simulink model "ControlR2019A"  (R2019a)
settings: Solver=FixedStepAuto  StartTime=0.0  StopTime=t_sim  FixedStep=TimeStep  RelTol=1e-3
values from neighbouring files (symbols this model uses):
  nmax = 2    [main_SCA.m]    (also in main_SCA_alt.m; main_SCA_v3.m)
  Use_IGRF = 0    [main_SCA.m]    (also in main_SCA_alt.m; main_SCA_v3.m)
undefined symbols (not defined in the file or in its folder): att, date, deg, DipoleMod, DiscIntNeverNeededParam, km, orbit, rad, s, sat
libraries: aerolibconvert2 x10, aerolibutil x10, vrlib x6, simulink x5, sharedtransform x4, dspmathops x4, sharedutil x2, dspstat3 x1, aerolibgravity2 x1, aerolibcelestial x1
(part 1 of 2)
settings Model: Creator=colpari  LastModifiedBy=colpari

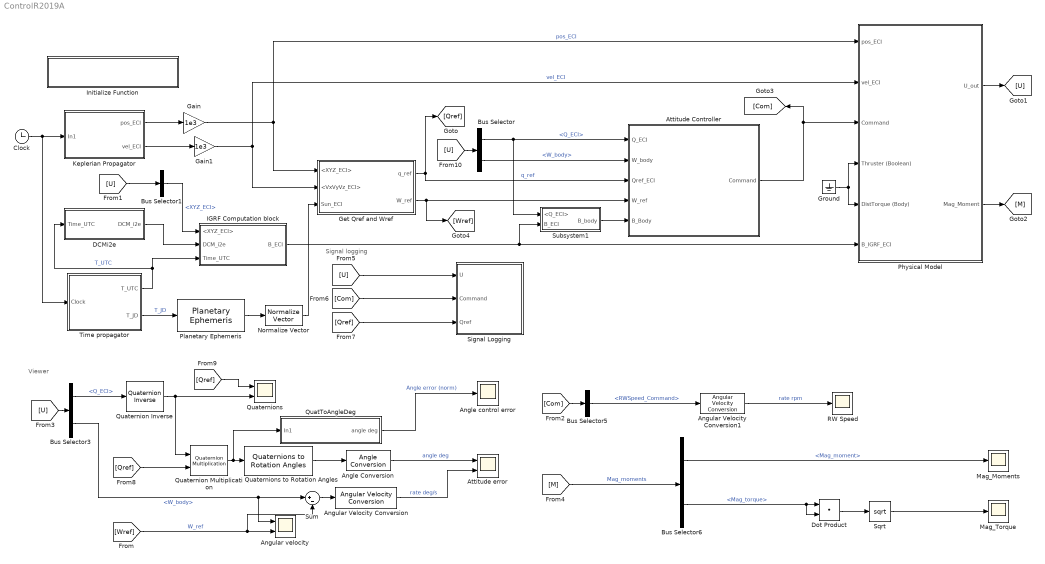
== system ControlR2019A ==
  note: Viewer
  note: Signal logging
  Angle Conversion : aerolibconvert2/Angle Conversion  IU=rad  OU=deg
  Angle control error : Scope
  Angular Velocity Conversion : aerolibconvert2/Angular Velocity Conversion  IU=rad/s  OU=deg/s
  Angular Velocity Conversion1 : aerolibconvert2/Angular Velocity Conversion  IU=rad/s  OU=rpm
  Angular velocity : Scope  NumInputPorts=2
  Attitude Controller : Subsystem  TreatAsAtomicUnit=on
  Attitude error : Scope  NumInputPorts=2
  Bus Selector : BusSelector  OutputSignals=Q_ECI,W_body
  Bus Selector1 : BusSelector  OutputSignals=XYZ_ECI
  Bus Selector3 : BusSelector  OutputSignals=Q_ECI,W_body
  Bus Selector5 : BusSelector  OutputSignals=RWSpeed_Command
  Bus Selector6 : BusSelector  OutputSignals=Mag_moment,Mag_torque
  Clock : Clock
  DCMi2e : Subsystem  TreatAsAtomicUnit=on  SystemSampleTime=1
  Dot Product : DotProduct  InputSameDT=on  OutDataTypeStr=Inherit: Inherit via internal rule
  Gain : Gain  Gain=1e3
  Gain1 : Gain  Gain=1e3
  Get Qref and Wref : Subsystem
  Ground : Ground
  IGRF Computation block : Subsystem
  Initialize Function : Subsystem  TreatAsAtomicUnit=on
  Keplerian Propagator : Subsystem
  Mag_Moments : Scope
  Mag_Torque : Scope
  Normalize Vector : vrlib/Utilities/Normalize Vector  maxzero=0
  Physical Model : Subsystem
      settings: MinAlgLoopOccurrences=on
  Planetary Ephemeris : aerolibcelestial/Planetary Ephemeris  kmflag=km,km/s  epochflag=Julian date  de=DE405  nCenter=Earth  nTarget=Sun  errorflag=Error  velflag=off
      settings: SourceProductBaseCode=AE
  QuatToAngleDeg : Subsystem
  Quaternion Inverse : aerolibutil/Quaternion Inverse
  Quaternion Multiplication : aerolibutil/Quaternion Multiplication
  Quaternions : Scope  NumInputPorts=2
  Quaternions to Rotation Angles : sharedtransform/Quaternions to Rotation Angles  rotationOrder=ZYX  aMode=aMode
      settings: SourceProductBaseCode=AE,PW,MT,UV,VE,VP
  RW Speed : Scope
  Signal Logging : Subsystem
  Sqrt : Sqrt  SaturateOnIntegerOverflow=on
  Subsystem1 : Subsystem
  Sum : Sum  Inputs=|+-
  Time propagator : Subsystem
  wires:
  Clock/1 -> Keplerian Propagator/1(In1), Time propagator/1(Clock)
  Keplerian Propagator/1(pos_ECI) -> Gain/1
  Keplerian Propagator/2(vel_ECI) -> Gain1/1
  Planetary Ephemeris/1 -> Normalize Vector/1
  Normalize Vector/1 -> Get Qref and Wref/3(Sun_ECI)
  Time propagator/2(T_JD) -> Planetary Ephemeris/1  "T_JD"
  Get Qref and Wref/1(q_ref) -> Attitude Controller/3(Qref_ECI), [Qref]  "q_ref"
  Physical Model/1(U_out) -> [U]
  Time propagator/1(T_UTC) -> DCMi2e/1(Time_UTC), IGRF Computation block/3("Time_UTC ")  "T_UTC"
  Gain/1 -> Physical Model/1(pos_ECI), Get Qref and Wref/1(<XYZ_ECI>)  "pos_ECI"
  Gain1/1 -> Physical Model/2(vel_ECI), Get Qref and Wref/2(<VxVyVz_ECI>)  "vel_ECI"
  DCMi2e/1(DCM_i2e) -> IGRF Computation block/2("DCM_i2e ")
  Attitude Controller/1(Command) -> [Com], Physical Model/3(Command)
  IGRF Computation block/1(B_ECI) -> Subsystem1/2(B_ECI), Physical Model/6(B_IGRF_ECI)
  [U] -> Bus Selector/1
  Bus Selector/1 -> Subsystem1/1(<Q_ECI>), Attitude Controller/1(Q_ECI)  "<Q_ECI>"
  Bus Selector/2 -> Attitude Controller/2(W_body)  "<W_body>"
  [U] -> Bus Selector1/1
  Bus Selector1/1 -> IGRF Computation block/1(<XYZ_ECI>)  "<XYZ_ECI>"
  [Qref] -> Signal Logging/3(Qref)
  Quaternions to Rotation Angles/1 -> Angle Conversion/1
  Bus Selector6/2 -> Dot Product/2, Dot Product/1  "<Mag_torque>"
  Bus Selector6/1 -> Mag_Moments/1  "<Mag_moment>"
  Dot Product/1 -> Sqrt/1
  Bus Selector3/1 -> Quaternion Inverse/1  "<Q_ECI>"
  Sqrt/1 -> Mag_Torque/1
  Bus Selector5/1 -> Angular Velocity Conversion1/1  "<RWSpeed_Command>"
  [Com] -> Signal Logging/2(Command)
  [Com] -> Bus Selector5/1
  Bus Selector3/2 -> Sum/1, Angular velocity/1  "<W_body>"
  [Qref] -> Quaternion Multiplication/2
  [U] -> Bus Selector3/1
  Quaternion Inverse/1 -> Quaternion Multiplication/1, Quaternions/2
  [M] -> Bus Selector6/1  "Mag_moments"
  Angular Velocity Conversion/1 -> Attitude error/2  "rate deg/s"
  Quaternion Multiplication/1 -> QuatToAngleDeg/1(In1), Quaternions to Rotation Angles/1
  [U] -> Signal Logging/1(U)
  Angle Conversion/1 -> Attitude error/1  "angle deg"
  Angular Velocity Conversion1/1 -> RW Speed/1  "rate rpm"
  Physical Model/2(Mag_Moment) -> [M]
  Subsystem1/1(B_body) -> Attitude Controller/5(B_Body)
  Ground/1 -> Physical Model/5(DistTorque (Body)), Physical Model/4(Thruster (Boolean))
  QuatToAngleDeg/1(angle deg) -> Angle control error/1  "Angle error (norm)"
  [Qref] -> Quaternions/1
  Get Qref and Wref/2(W_ref) -> [Wref], Attitude Controller/4(W_ref)
  [Wref] -> Sum/2, Angular velocity/2  "W_ref"
  Sum/1 -> Angular Velocity Conversion/1

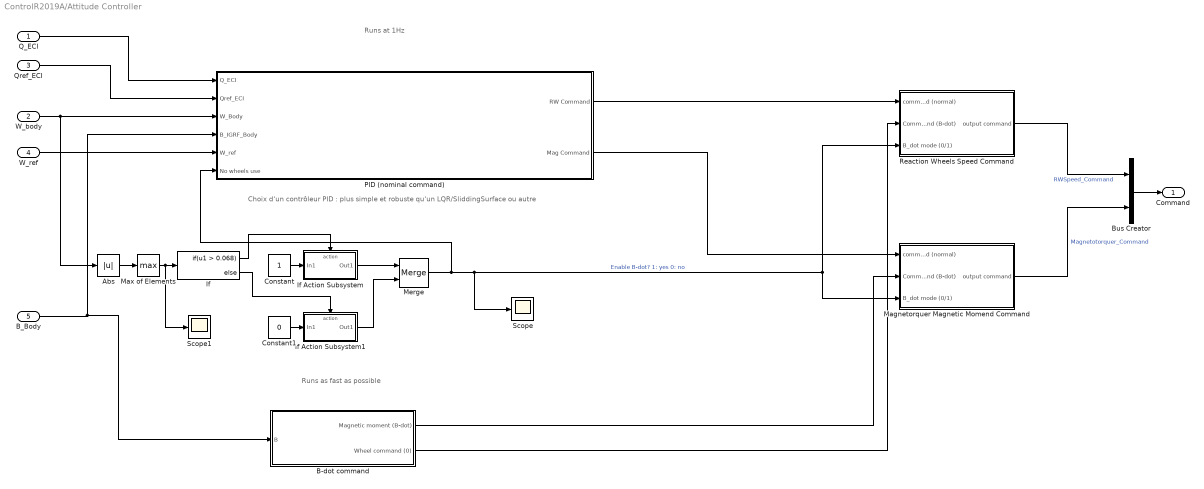
== system ControlR2019A/Attitude Controller ==
  note: Choix d'un contrôleur PID : plus simple et robuste qu'un LQR/SliddingSurface ou autre
  note: Runs as fast as possible
  note: Runs at 1Hz
  Q_ECI : Inport
  W_body : Inport  Port=2
  Qref_ECI : Inport  Port=3
  W_ref : Inport  Port=4
  B_Body : Inport  Port=5
  Abs : Abs
  B-dot command : Subsystem  TreatAsAtomicUnit=on
  Bus Creator : BusCreator  Inputs=2
  Constant : Constant
  Constant1 : Constant  Value=0
  If : If  IfExpression=u1 > 0.068
  If Action Subsystem : Subsystem  TreatAsAtomicUnit=on
  If Action Subsystem1 : Subsystem  TreatAsAtomicUnit=on
  Magnetorquer Magnetic Momend Command : Subsystem
  Max of Elements : MinMax  Function=max
  Merge : Merge
  PID (nominal command) : Subsystem  TreatAsAtomicUnit=on  SystemSampleTime=1
  Reaction Wheels Speed Command : Subsystem
  Scope : Scope
  Scope1 : Scope
  Command : Outport  VectorParamsAs1DForOutWhenUnconnected=off
  wires:
  B_Body/1 -> B-dot command/1(B), PID (nominal command)/4(B_IGRF_Body)
  Magnetorquer Magnetic Momend Command/1(output command) -> Bus Creator/2  "Magnetotorquer_Command"
  Reaction Wheels Speed Command/1(output command) -> Bus Creator/1  "RWSpeed_Command"
  B-dot command/2(Wheel command (0)) -> Reaction Wheels Speed Command/2(Command (B-dot))
  B-dot command/1(Magnetic moment (B-dot)) -> Magnetorquer Magnetic Momend Command/2(Command (B-dot))
  Q_ECI/1 -> PID (nominal command)/1(Q_ECI)
  Qref_ECI/1 -> PID (nominal command)/2(Qref_ECI)
  PID (nominal command)/1(RW Command) -> Reaction Wheels Speed Command/1(" command (normal)")
  PID (nominal command)/2(Mag Command) -> Magnetorquer Magnetic Momend Command/1(" command (normal)")
  Bus Creator/1 -> Command/1
  Abs/1 -> Max of Elements/1
  If/1 -> If Action Subsystem/Action
  If Action Subsystem1/1(Out1) -> Merge/2
  Max of Elements/1 -> Scope1/1, If/1
  If/2 -> If Action Subsystem1/Action
  If Action Subsystem/1(Out1) -> Merge/1
  Constant/1 -> If Action Subsystem/1(In1)
  Merge/1 -> Scope/1, Magnetorquer Magnetic Momend Command/3(B_dot mode (0/1)), Reaction Wheels Speed Command/3(B_dot mode (0/1)), PID (nominal command)/6(No wheels use)  "Enable B-dot? 1: yes 0: no"
  Constant1/1 -> If Action Subsystem1/1(In1)
  W_body/1 -> Abs/1, PID (nominal command)/3(W_Body)
  W_ref/1 -> PID (nominal command)/5(W_ref)

== system ControlR2019A/DCMi2e ==
  note: Slower subsytem because it's too slow
  Time_UTC : Inport
  ECI to ECEF : MATLABFcn  MATLABFcn=eci2ecef  OutputDimensions=[3;3]  Output1D=off
  DCM_i2e : Outport
  wires:
  ECI to ECEF/1 -> DCM_i2e/1
  Time_UTC/1 -> ECI to ECEF/1

== system ControlR2019A/Get Qref and Wref ==
  <XYZ_ECI> : Inport
  <VxVyVz_ECI> : Inport  Port=2
  Sun_ECI : Inport  Port=3
  Manual Switch : ManualSwitch  CurrentSetting=0
  Manual Switch1 : ManualSwitch  CurrentSetting=0
  Scope : Scope  NumInputPorts=2
  q_orbital : Subsystem
  q_sun_aero : Subsystem
  q_ref : Outport
  W_ref : Outport  Port=2
  wires:
  q_sun_aero/1(Q_sun_aero) -> Manual Switch/2
  <VxVyVz_ECI>/1 -> q_sun_aero/2(<VxVyVz_ECI>), q_orbital/2(<VxVyVz_ECI>)
  q_orbital/1(Q_orbit) -> Manual Switch/1
  Sun_ECI/1 -> q_sun_aero/1(Sun_ECI)
  <XYZ_ECI>/1 -> q_orbital/1(<XYZ_ECI>)
  Manual Switch/1 -> q_ref/1, Scope/1
  Manual Switch1/1 -> Scope/2, W_ref/1
  q_sun_aero/2(W_sun_aero) -> Manual Switch1/2
  q_orbital/2(W_orbit) -> Manual Switch1/1

== system ControlR2019A/IGRF Computation block ==
  <XYZ_ECI> : Inport
  "DCM_i2e " : Inport  Port=2
  "Time_UTC " : Inport  Port=3
  Bus Creator : BusCreator  Inputs=5
  Bus Selector4 : BusSelector  OutputSignals=XYZ_ECI
  Demux : Demux  Outputs=2
  ECI To LLA : MATLAB Function  TreatAsAtomicUnit=on
  Obtain B_ECI : Subsystem
  Product : Product  Multiplication=Matrix(*)
  Reshape : Reshape  OutputDimensionality=Row vector (2-D)
  Terminator : Terminator
  B_ECI : Outport  VectorParamsAs1DForOutWhenUnconnected=off
  wires:
  ECI To LLA/3(long) -> Bus Creator/3
  ECI To LLA/2(lat) -> Bus Creator/2
  ECI To LLA/1(h) -> Bus Creator/1
  Demux/1 -> Bus Creator/4
  Demux/2 -> Terminator/1
  "DCM_i2e "/1 -> Product/2, Bus Creator/5  "DCM_i2e"
  <XYZ_ECI>/1 -> Bus Selector4/1
  Reshape/1 -> Product/1
  Product/1 -> ECI To LLA/1(X_ECEF)
  Bus Selector4/1 -> Reshape/1  "<XYZ_ECI>"
  Bus Creator/1 -> Obtain B_ECI/1(In1)
  Obtain B_ECI/1(Out1) -> B_ECI/1
  "Time_UTC "/1 -> Demux/1

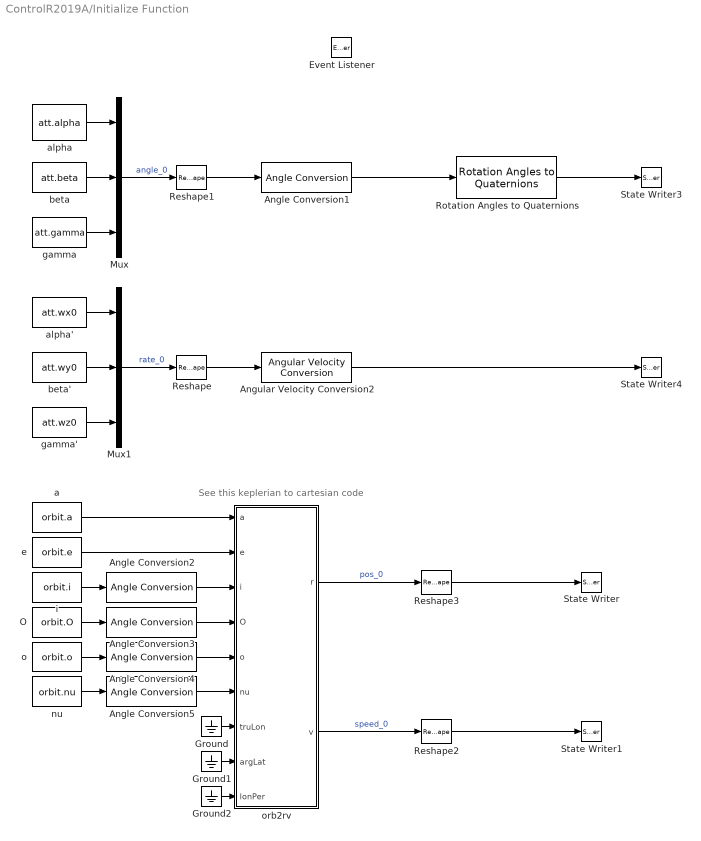
== system ControlR2019A/Initialize Function ==
  note: See this keplerian to cartesian code
  Angle Conversion{1..5} (5 alike) : aerolibconvert2/Angle Conversion  IU=deg  OU=rad
  Angular Velocity Conversion2 : aerolibconvert2/Angular Velocity Conversion  IU=deg/s  OU=rad/s
  Event Listener : EventListener  DisableCoverage=on  EventName=reset
  Ground : Ground
  Ground1 : Ground
  Ground2 : Ground
  Mux : Mux  Inputs=3
  Mux1 : Mux  Inputs=3
  O : Constant  Value=orbit.O
  Reshape{,1..3} (4 alike) : Reshape  OutputDimensionality=Column vector (2-D)
  Rotation Angles to Quaternions : sharedtransform/Rotation Angles to Quaternions  rotationOrder=ZYX  aMode=aMode
      settings: SourceProductBaseCode=AE,PW,MT,UV,VE,VP
  State Writer : StateWriter  StateOwnerBlock=../../Keplerian Propagator/Integrator
  State Writer1 : StateWriter  StateOwnerBlock=../../Keplerian Propagator/Integrator1
  State Writer3 : StateWriter  StateOwnerBlock=../../Physical Model/6DOF in ECI frame/Compute Q_ECI/Integrator_quat
  State Writer4 : StateWriter  StateOwnerBlock=../../Physical Model/6DOF in ECI frame/Integrator_rate
  a : Constant  Value=orbit.a
  alpha : Constant  Value=att.alpha
  alpha' : Constant  Value=att.wx0
  beta : Constant  Value=att.beta
  beta' : Constant  Value=att.wy0
  e : Constant  Value=orbit.e
  gamma : Constant  Value=att.gamma
  gamma' : Constant  Value=att.wz0
  i : Constant  Value=orbit.i
  nu : Constant  Value=orbit.nu
  o : Constant  Value=orbit.o
  orb2rv : MATLAB Function  TreatAsAtomicUnit=on
  wires:
  Angular Velocity Conversion2/1 -> State Writer4/1
  Angle Conversion1/1 -> Rotation Angles to Quaternions/1
  Mux1/1 -> Reshape/1  "rate_0"
  Mux/1 -> Reshape1/1  "angle_0"
  Rotation Angles to Quaternions/1 -> State Writer3/1
  Reshape/1 -> Angular Velocity Conversion2/1
  Reshape1/1 -> Angle Conversion1/1
  alpha/1 -> Mux/1
  beta/1 -> Mux/2
  gamma/1 -> Mux/3
  alpha'/1 -> Mux1/1
  gamma'/1 -> Mux1/3
  beta'/1 -> Mux1/2
  Reshape2/1 -> State Writer1/1
  Reshape3/1 -> State Writer/1
  i/1 -> Angle Conversion2/1
  Ground/1 -> orb2rv/7(truLon)
  Angle Conversion2/1 -> orb2rv/3(i)
  nu/1 -> Angle Conversion5/1
  Ground2/1 -> orb2rv/9(lonPer)
  Angle Conversion3/1 -> orb2rv/4(O)
  Angle Conversion5/1 -> orb2rv/6(nu)
  Ground1/1 -> orb2rv/8(argLat)
  o/1 -> Angle Conversion4/1
  a/1 -> orb2rv/1(a)
  O/1 -> Angle Conversion3/1
  orb2rv/2(v) -> Reshape2/1  "speed_0"
  e/1 -> orb2rv/2(e)
  orb2rv/1(r) -> Reshape3/1  "pos_0"
  Angle Conversion4/1 -> orb2rv/5(o)

== system ControlR2019A/Keplerian Propagator ==
  In1 : Inport
  Constant : Constant  Value=[0;0;0]
  Demux : Demux  Outputs=2
  Integrator : Integrator
  Integrator1 : Integrator
  Mux : Mux  Inputs=2
  Mux1 : Mux  Inputs=2
  Reshape1 : Reshape  OutputDimensionality=Customize  OutputDimensions=[6,1]
  Reshape3 : Reshape  OutputDimensionality=Column vector (2-D)
  keplerian propagator : MATLABFcn  MATLABFcn=kep_propagator
  pos_ECI : Outport
  vel_ECI : Outport  Port=2
  wires:
  Demux/2 -> vel_ECI/1  "vel_ECI"
  Demux/1 -> pos_ECI/1  "pos_ECI"
  keplerian propagator/1 -> Demux/1
  Mux1/1 -> keplerian propagator/1
  In1/1 -> Mux1/2
  Mux/1 -> Reshape1/1
  Reshape1/1 -> Mux1/1
  Integrator1/1 -> Mux/2
  Constant/1 -> Reshape3/1
  Reshape3/1 -> Integrator1/1, Integrator/1
  Integrator/1 -> Mux/1

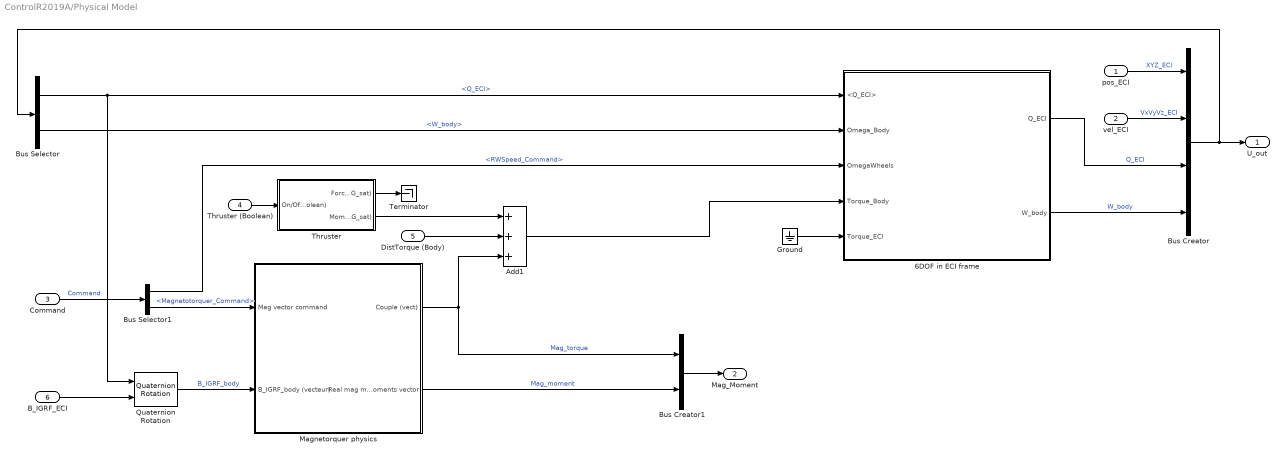
== system ControlR2019A/Physical Model ==
  pos_ECI : Inport
  vel_ECI : Inport  Port=2
  Command : Inport  Port=3
  Thruster (Boolean) : Inport  Port=4
  DistTorque (Body) : Inport  Port=5
  B_IGRF_ECI : Inport  Port=6
  6DOF in ECI frame : Subsystem
  Add1 : Sum  Inputs=+++
  Bus Creator : BusCreator  Inputs=4
  Bus Creator1 : BusCreator  Inputs=2
  Bus Selector : BusSelector  OutputSignals=Q_ECI,W_body
  Bus Selector1 : BusSelector  OutputSignals=RWSpeed_Command,Magnetotorquer_Command
  Ground : Ground
  Magnetorquer physics : Subsystem
  Quaternion Rotation : aerolibutil/Quaternion Rotation
  Terminator : Terminator
  Thruster : Subsystem
  U_out : Outport  VectorParamsAs1DForOutWhenUnconnected=off
  Mag_Moment : Outport  Port=2  VectorParamsAs1DForOutWhenUnconnected=off
  wires:
  Thruster (Boolean)/1 -> Thruster/1(On/Off (Boolean))
  Bus Creator/1 -> U_out/1, Bus Selector/1
  Bus Selector/1 -> Quaternion Rotation/1, 6DOF in ECI frame/1(<Q_ECI>)  "<Q_ECI>"
  6DOF in ECI frame/1(Q_ECI) -> Bus Creator/3  "Q_ECI"
  Bus Selector1/2 -> Magnetorquer physics/1(Mag vector command)  "<Magnetotorquer_Command>"
  Thruster/2(Moment (G_sat)) -> Add1/1
  Add1/1 -> 6DOF in ECI frame/4(Torque_Body)
  DistTorque (Body)/1 -> Add1/2
  Bus Selector/2 -> 6DOF in ECI frame/2("Omega_Body ")  "<W_body>"
  B_IGRF_ECI/1 -> Quaternion Rotation/2
  Quaternion Rotation/1 -> Magnetorquer physics/2(B_IGRF_body (vecteur))  "B_IGRF_body"
  Magnetorquer physics/2(Real mag moments vector) -> Bus Creator1/2  "Mag_moment"
  Magnetorquer physics/1(Couple (vect)) -> Add1/3, Bus Creator1/1  "Mag_torque"
  6DOF in ECI frame/2(W_body) -> Bus Creator/4  "W_body"
  Command/1 -> Bus Selector1/1  "Command"
  Bus Selector1/1 -> 6DOF in ECI frame/3(OmegaWheels)  "<RWSpeed_Command>"
  Bus Creator1/1 -> Mag_Moment/1
  pos_ECI/1 -> Bus Creator/1  "XYZ_ECI"
  vel_ECI/1 -> Bus Creator/2  "VxVyVz_ECI"
  Thruster/1(Force (G_sat)) -> Terminator/1
  Ground/1 -> 6DOF in ECI frame/5(Torque_ECI)

== system ControlR2019A/QuatToAngleDeg ==
  In1 : Inport
  Abs : Abs
  Angle Conversion1 : aerolibconvert2/Angle Conversion  IU=rad  OU=deg
  Demux1 : Demux
  Quaternion to axis and angle conversion : MATLABFcn  MATLABFcn=quat2axisangle
  Terminator1 : Terminator
  Terminator2 : Terminator
  Terminator3 : Terminator
  angle deg : Outport  VectorParamsAs1DForOutWhenUnconnected=off
  wires:
  Demux1/2 -> Terminator2/1
  Demux1/4 -> Angle Conversion1/1
  In1/1 -> Quaternion to axis and angle conversion/1
  Demux1/1 -> Terminator1/1
  Demux1/3 -> Terminator3/1
  Quaternion to axis and angle conversion/1 -> Demux1/1
  Abs/1 -> angle deg/1
  Angle Conversion1/1 -> Abs/1  "angle deg"

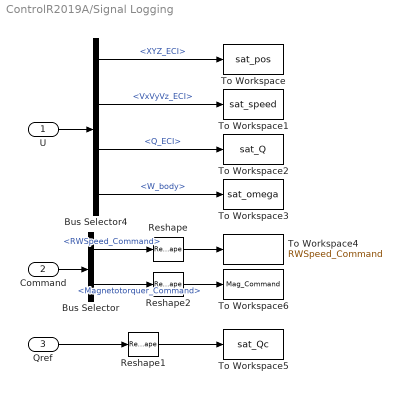
== system ControlR2019A/Signal Logging ==
  U : Inport
  Command : Inport  Port=2
  Qref : Inport  Port=3
  Bus Selector : BusSelector  OutputSignals=RWSpeed_Command,Magnetotorquer_Command
  Bus Selector4 : BusSelector  OutputSignals=XYZ_ECI,VxVyVz_ECI,Q_ECI,W_body
  Reshape : Reshape
  Reshape1 : Reshape
  Reshape2 : Reshape
  To Workspace : ToWorkspace  VariableName=sat_pos  SaveFormat=Timeseries  SampleTime=1
      settings: Save2DSignal=2-D array (concatenate along first dimension)
  To Workspace1 : ToWorkspace  VariableName=sat_speed  SaveFormat=Timeseries  SampleTime=1
      settings: Save2DSignal=2-D array (concatenate along first dimension)
  To Workspace2 : ToWorkspace  VariableName=sat_Q  SaveFormat=Timeseries  SampleTime=1
      settings: Save2DSignal=2-D array (concatenate along first dimension)
  To Workspace3 : ToWorkspace  VariableName=sat_omega  SaveFormat=Timeseries  SampleTime=1
      settings: Save2DSignal=2-D array (concatenate along first dimension)
  To Workspace4 : ToWorkspace  VariableName=RWSpeed_Command  SaveFormat=Timeseries  SampleTime=1
      settings: Save2DSignal=2-D array (concatenate along first dimension)
  To Workspace5 : ToWorkspace  VariableName=sat_Qc  SaveFormat=Timeseries  SampleTime=1
      settings: Save2DSignal=2-D array (concatenate along first dimension)
  To Workspace6 : ToWorkspace  VariableName=Mag_Command  SaveFormat=Timeseries  SampleTime=1
      settings: Save2DSignal=2-D array (concatenate along first dimension)
  wires:
  Bus Selector4/3 -> To Workspace2/1  "<Q_ECI>"
  Bus Selector4/4 -> To Workspace3/1  "<W_body>"
  U/1 -> Bus Selector4/1
  Bus Selector4/2 -> To Workspace1/1  "<VxVyVz_ECI>"
  Command/1 -> Bus Selector/1
  Bus Selector4/1 -> To Workspace/1  "<XYZ_ECI>"
  Qref/1 -> Reshape1/1
  Reshape/1 -> To Workspace4/1
  Reshape1/1 -> To Workspace5/1
  Bus Selector/1 -> Reshape/1  "<RWSpeed_Command>"
  Bus Selector/2 -> Reshape2/1  "<Magnetotorquer_Command>"
  Reshape2/1 -> To Workspace6/1

== system ControlR2019A/Subsystem1 ==
  <Q_ECI> : Inport
  B_ECI : Inport  Port=2
  Quaternion Rotation : aerolibutil/Quaternion Rotation
  B_body : Outport
  wires:
  <Q_ECI>/1 -> Quaternion Rotation/1
  B_ECI/1 -> Quaternion Rotation/2
  Quaternion Rotation/1 -> B_body/1  "B_IGRF_body"

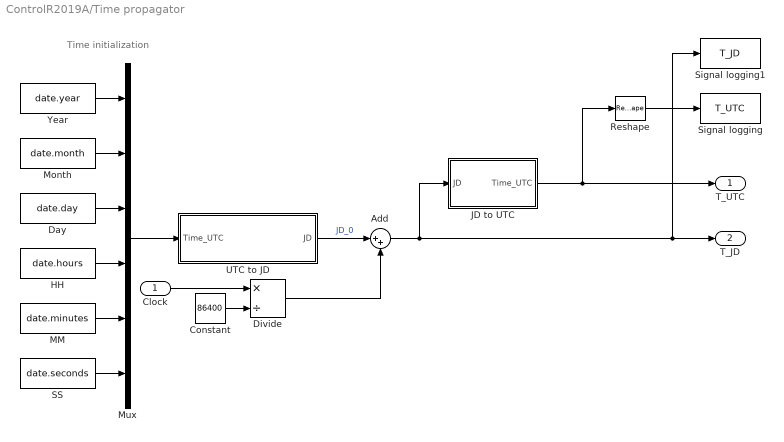
== system ControlR2019A/Time propagator ==
  note: Time initialization
  Clock : Inport
  Add : Sum  Inputs=|++
  Constant : Constant  Value=86400
  Day : Constant  Value=date.day
  Divide : Product  Inputs=*/
  HH : Constant  Value=date.hours
  JD to UTC : MATLAB Function  TreatAsAtomicUnit=on
  MM : Constant  Value=date.minutes
  Month : Constant  Value=date.month
  Mux : Mux  Inputs=6
  Reshape : Reshape
  SS : Constant  Value=date.seconds
  Signal logging : ToWorkspace  VariableName=T_UTC  SaveFormat=Timeseries  SampleTime=1
      settings: Save2DSignal=2-D array (concatenate along first dimension)
  Signal logging1 : ToWorkspace  VariableName=T_JD  SaveFormat=Timeseries  SampleTime=1
      settings: Save2DSignal=2-D array (concatenate along first dimension)
  UTC to JD : MATLAB Function  TreatAsAtomicUnit=on
  Year : Constant  Value=date.year
  T_UTC : Outport  VectorParamsAs1DForOutWhenUnconnected=off
  T_JD : Outport  Port=2  VectorParamsAs1DForOutWhenUnconnected=off
  wires:
  UTC to JD/1(JD) -> Add/1  "JD_0"
  Clock/1 -> Divide/1
  Constant/1 -> Divide/2
  JD to UTC/1(Time_UTC) -> T_UTC/1, Reshape/1
  Divide/1 -> Add/2
  Mux/1 -> UTC to JD/1(Time_UTC)
  Day/1 -> Mux/3
  Month/1 -> Mux/2
  Year/1 -> Mux/1
  HH/1 -> Mux/4
  MM/1 -> Mux/5
  SS/1 -> Mux/6
  Reshape/1 -> Signal logging/1
  Add/1 -> Signal logging1/1, T_JD/1, JD to UTC/1(JD)

== system ControlR2019A/Attitude Controller/B-dot command ==
  note: ref : OneDrive\IonSat X18\SCAO\Contrôle attitude\Detumbling\Detumbling and Aerostable Control for Cubesats.pdf
      |
      | formulae:
      | $\mathbf{\dot B} \simeq \mathbf{B}\times \mathbf{\dot \theta}$
      | $\mathbf{m} = -c\mathbf{\dot B}$
      |
      | this block does NOT decide if the B-dot mode is relevant or not
      | (it applies it without question on the rotation rate :
      | $\Omega=v/r= \sqrt{\frac{Gm_{earth}}{(h+r_{earth})^{3/2}}} \sim 0.066 °/s$ So the command MUST stop the B-dot mode when the estimated rotation speed is smaller than 0.1 degree per second )
  note: entrée:
      | champ magnétique
      | sortie: moment magnetique de commande et vitesse des roues à réaction (nulle)
  B : Inport
  Discrete Derivative : simulink/Discrete/Discrete Derivative  gainval=1.0  ICPrevScaledInput=0.0  OutMin=[]  OutMax=[]  OutDataType=fixdt(1, 16)  OutScaling=2^-10  DoSatur=off
  Divide1 : Product  Inputs=**
  Reshape2 : Reshape  OutputDimensionality=Column vector (2-D)
  constant c : Constant  Value=-sat.bdot_c
  wheels unused : Constant  Value=[0, 0, 0, 0]
  Magnetic moment (B-dot) : Outport  VectorParamsAs1DForOutWhenUnconnected=off
  Wheel command (0) : Outport  Port=2  VectorParamsAs1DForOutWhenUnconnected=off
  wires:
  constant c/1 -> Divide1/2
  B/1 -> Discrete Derivative/1
  Discrete Derivative/1 -> Divide1/1  "B_point=B^theta_point"
  Divide1/1 -> Magnetic moment (B-dot)/1
  wheels unused/1 -> Reshape2/1
  Reshape2/1 -> Wheel command (0)/1

== system ControlR2019A/Attitude Controller/If Action Subsystem ==
  In1 : Inport
  Action Port : ActionPort
  Out1 : Outport  VectorParamsAs1DForOutWhenUnconnected=off
  wires:
  In1/1 -> Out1/1

== system ControlR2019A/Attitude Controller/If Action Subsystem1 ==
  In1 : Inport
  Action Port : ActionPort
  Out1 : Outport  VectorParamsAs1DForOutWhenUnconnected=off
  wires:
  In1/1 -> Out1/1

== system ControlR2019A/Attitude Controller/Magnetorquer Magnetic Momend Command ==
  " command (normal)" : Inport
  Command (B-dot) : Inport  Port=2
  B_dot mode (0/1) : Inport  Port=3
  If1 : If
  Merge : Merge
  Switch Case Action Subsystem3 : Subsystem  TreatAsAtomicUnit=on
  Switch Case Action Subsystem4 : Subsystem  TreatAsAtomicUnit=on
  output command : Outport  VectorParamsAs1DForOutWhenUnconnected=off
  wires:
  If1/2 -> Switch Case Action Subsystem4/Action
  If1/1 -> Switch Case Action Subsystem3/Action
  B_dot mode (0/1)/1 -> If1/1
  Command (B-dot)/1 -> Switch Case Action Subsystem3/1(In1)
  Switch Case Action Subsystem3/1(Out1) -> Merge/1
  Switch Case Action Subsystem4/1(Out1) -> Merge/2
  " command (normal)"/1 -> Switch Case Action Subsystem4/1(In1)
  Merge/1 -> output command/1

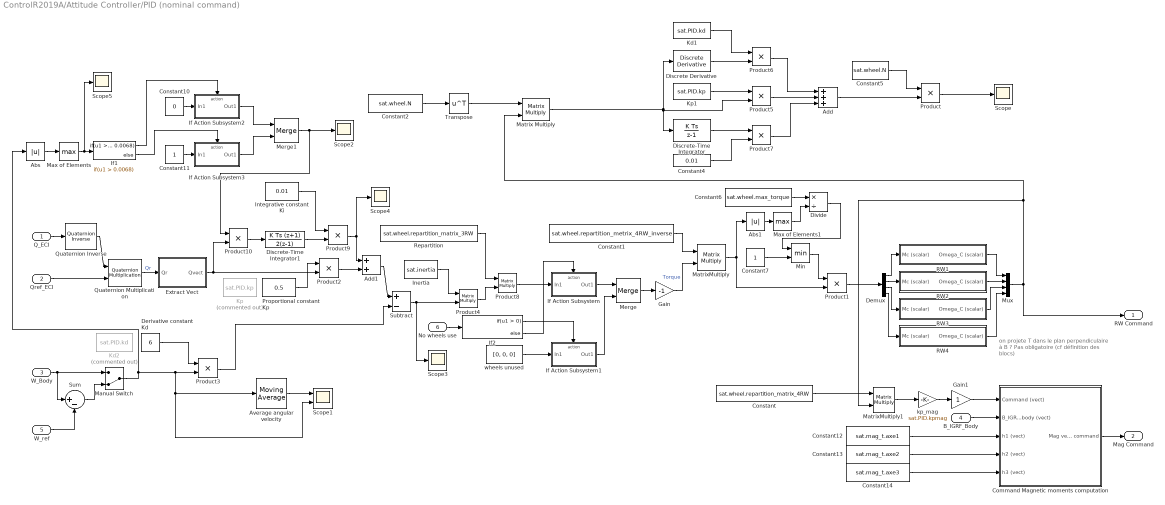
== system ControlR2019A/Attitude Controller/PID (nominal command) ==
  note: on projete T dans
      | le plan perpendiculaire à B ?
      | Pas obligatoire (cf définition des blocs)
  Q_ECI : Inport
  Qref_ECI : Inport  Port=2
  W_Body : Inport  Port=3
  B_IGRF_Body : Inport  Port=4
  W_ref : Inport  Port=5
  No wheels use : Inport  Port=6
  Abs : Abs
  Abs1 : Abs
  Add : Sum  Inputs=+++
  Add1 : Sum
  Average angular velocity : dspstat3/Moving Average  Method=Sliding window  ForgettingFactorPort=off  SpecifyWindowLength=on  WindowLength=4  ForgettingFactor=0.9  SimulateUsing=Code generation
  Command Magnetic moments computation : Subsystem
  Constant : Constant  Value=sat.wheel.repartition_matrix_4RW
  Constant1 : Constant  Value=sat.wheel.repartition_metrix_4RW_inverse
  Constant10 : Constant  Value=0
  Constant11 : Constant
  Constant12 : Constant  Value=sat.mag_t.axe1
  Constant13 : Constant  Value=sat.mag_t.axe2
  Constant14 : Constant  Value=sat.mag_t.axe3
  Constant2 : Constant  Value=sat.wheel.N
  Constant4 : Constant  Value=0.01
  Constant5 : Constant  Value=sat.wheel.N
  Constant6 : Constant  Value=sat.wheel.max_torque
  Constant7 : Constant
  Demux : Demux
  Derivative constant Kd : Constant  Value=6
  Discrete Derivative : simulink/Discrete/Discrete Derivative  gainval=1.0  ICPrevScaledInput=0.0  OutMin=[]  OutMax=[]  OutDataType=fixdt(1, 16)  OutScaling=2^-10  DoSatur=off
  Discrete-Time Integrator : DiscreteIntegrator  SampleTime=-1  ICPrevOutput=DiscIntNeverNeededParam  ICPrevScaledInput=DiscIntNeverNeededParam
  Discrete-Time Integrator1 : DiscreteIntegrator  IntegratorMethod=Integration: Trapezoidal  SampleTime=-1  ICPrevOutput=DiscIntNeverNeededParam  ICPrevScaledInput=DiscIntNeverNeededParam
  Divide : Product  Inputs=*/
  Extract Vect : Subsystem
  Gain : Gain  Gain=-1
  Gain1 : Gain
  If Action Subsystem : Subsystem  TreatAsAtomicUnit=on
  If Action Subsystem1 : Subsystem  TreatAsAtomicUnit=on
  If Action Subsystem2 : Subsystem  TreatAsAtomicUnit=on
  If Action Subsystem3 : Subsystem  TreatAsAtomicUnit=on
  If1 : If  IfExpression=u1 > 0.0068
  If2 : If
  Inertia : Constant  Value=sat.inertia
  Integrative constant Ki : Constant  Value=0.01
  Kd1 : Constant  Value=sat.PID.kd
  Kd2 : Constant  Commented=on  Value=sat.PID.kd
  Kp : Constant  Commented=on  Value=sat.PID.kp
  Kp1 : Constant  Value=sat.PID.kp
  Manual Switch : ManualSwitch  CurrentSetting=0
  Matrix Multiply : Product  Multiplication=Matrix(*)
  MatrixMultiply : Product  Multiplication=Matrix(*)
  MatrixMultiply1 : Product  Multiplication=Matrix(*)
  Max of Elements : MinMax  Function=max
  Max of Elements1 : MinMax  Function=max
  Merge : Merge
  Merge1 : Merge
  Min : MinMax  Inputs=2
  Mux : Mux
  Product{,1..3,5..7,9..10} (9 alike) : Product
  Product4 : Product  Multiplication=Matrix(*)
  Product8 : Product  Multiplication=Matrix(*)
  Proportional constant Kp : Constant  Value=0.5
  Quaternion Inverse : aerolibutil/Quaternion Inverse
  Quaternion Multiplication : aerolibutil/Quaternion Multiplication
  RW1 : Subsystem
  RW2 : Subsystem
  RW3 : Subsystem
  "RW4 " : Subsystem
  Repartition : Constant  Value=sat.wheel.repartition_matrix_3RW
  Scope{,2..5} (5 alike) : Scope
  Scope1 : Scope  NumInputPorts=2
  Subtract : Sum  Inputs=+-
  Sum : Sum  Inputs=|+-
  Transpose : Math  Operator=transpose  SaturateOnIntegerOverflow=on
  kp_mag : Gain  Gain=sat.PID.kpmag
  wheels unused : Constant  Value=[0, 0, 0]
  RW Command : Outport  VectorParamsAs1DForOutWhenUnconnected=off
  Mag Command : Outport  Port=2  VectorParamsAs1DForOutWhenUnconnected=off
  wires:
  Constant2/1 -> Transpose/1
  Kp1/1 -> Product5/1
  Discrete Derivative/1 -> Product6/2
  Kd1/1 -> Product6/1
  Discrete-Time Integrator/1 -> Product7/1
  Constant4/1 -> Product7/2
  Product6/1 -> Add/1
  Product5/1 -> Add/2
  Product7/1 -> Add/3
  Constant5/1 -> Product/1
  Add/1 -> Product/2
  Matrix Multiply/1 -> Discrete-Time Integrator/1, Product5/2, Discrete Derivative/1
  Transpose/1 -> Matrix Multiply/1
  Product/1 -> Scope/1
  No wheels use/1 -> If2/1
  MatrixMultiply/1 -> Abs1/1, Product1/2
  Command Magnetic moments computation/1(Mag vector command) -> Mag Command/1
  Merge/1 -> Gain/1
  Product8/1 -> If Action Subsystem/1(In1)
  Constant14/1 -> Command Magnetic moments computation/5(h3 (vect))
  Constant12/1 -> Command Magnetic moments computation/3(h1 (vect))
  Constant/1 -> MatrixMultiply1/1
  Manual Switch/1 -> Abs/1, Scope1/2, Average angular velocity/1, Product3/2
  Constant11/1 -> If Action Subsystem3/1(In1)
  If2/2 -> If Action Subsystem/Action
  Max of Elements1/1 -> Divide/2
  Abs1/1 -> Max of Elements1/1
  Average angular velocity/1 -> Scope1/1
  Product10/1 -> Discrete-Time Integrator1/1
  Constant10/1 -> If Action Subsystem2/1(In1)
  Derivative constant Kd/1 -> Product3/1
  Demux/4 -> "RW4 "/1(Mc (scalar))
  Constant6/1 -> Divide/1
  Constant13/1 -> Command Magnetic moments computation/4(h2 (vect))
  Add1/1 -> Subtract/1
  Abs/1 -> Max of Elements/1
  Demux/3 -> RW3/1(Mc (scalar))
  Inertia/1 -> Product4/1
  RW3/1(Omega_C (scalar)) -> Mux/3
  Product9/1 -> Scope4/1, Add1/1
  RW2/1(Omega_C (scalar)) -> Mux/2
  Demux/2 -> RW2/1(Mc (scalar))
  RW1/1(Omega_C (scalar)) -> Mux/1
  Demux/1 -> RW1/1(Mc (scalar))
  If Action Subsystem/1(Out1) -> Merge/1
  Mux/1 -> Matrix Multiply/2, MatrixMultiply1/2, RW Command/1
  If1/2 -> If Action Subsystem3/Action
  Constant7/1 -> Min/2
  If Action Subsystem3/1(Out1) -> Merge1/2
  If Action Subsystem2/1(Out1) -> Merge1/1
  Subtract/1 -> Scope3/1, Product4/2
  Repartition/1 -> Product8/1
  Gain1/1 -> Command Magnetic moments computation/1(Command (vect))
  Constant1/1 -> MatrixMultiply/1
  Divide/1 -> Min/1
  Qref_ECI/1 -> Quaternion Multiplication/2
  wheels unused/1 -> If Action Subsystem1/1(In1)
  Max of Elements/1 -> Scope5/1, If1/1
  Merge1/1 -> Scope2/1, Product10/1
  Product4/1 -> Product8/2
  B_IGRF_Body/1 -> Command Magnetic moments computation/2(B_IGRF_body (vect))
  Q_ECI/1 -> Quaternion Inverse/1
  Product2/1 -> Add1/2
  "RW4 "/1(Omega_C (scalar)) -> Mux/4
  Discrete-Time Integrator1/1 -> Product9/2
  Proportional constant Kp/1 -> Product2/1
  If1/1 -> If Action Subsystem2/Action
  If2/1 -> If Action Subsystem1/Action
  Quaternion Multiplication/1 -> Extract Vect/1(Qr)  "Qr"
  Extract Vect/1(Qvect) -> Product10/2, Product2/2
  Min/1 -> Product1/1
  Integrative constant Ki/1 -> Product9/1
  If Action Subsystem1/1(Out1) -> Merge/2
  Product1/1 -> Demux/1
  Product3/1 -> Subtract/2
  kp_mag/1 -> Gain1/1
  Quaternion Inverse/1 -> Quaternion Multiplication/1
  MatrixMultiply1/1 -> kp_mag/1
  Gain/1 -> MatrixMultiply/2  "Torque"
  W_Body/1 -> Sum/1, Manual Switch/1
  W_ref/1 -> Sum/2
  Sum/1 -> Manual Switch/2

== system ControlR2019A/Attitude Controller/Reaction Wheels Speed Command ==
  " command (normal)" : Inport
  Command (B-dot) : Inport  Port=2
  B_dot mode (0/1) : Inport  Port=3
  If1 : If
  Merge : Merge
  Switch Case Action Subsystem3 : Subsystem  TreatAsAtomicUnit=on
  Switch Case Action Subsystem4 : Subsystem  TreatAsAtomicUnit=on
  output command : Outport  VectorParamsAs1DForOutWhenUnconnected=off
  wires:
  If1/2 -> Switch Case Action Subsystem4/Action
  If1/1 -> Switch Case Action Subsystem3/Action
  B_dot mode (0/1)/1 -> If1/1
  Command (B-dot)/1 -> Switch Case Action Subsystem3/1(In1)
  Merge/1 -> output command/1
  Switch Case Action Subsystem3/1(Out1) -> Merge/1
  Switch Case Action Subsystem4/1(Out1) -> Merge/2
  " command (normal)"/1 -> Switch Case Action Subsystem4/1(In1)

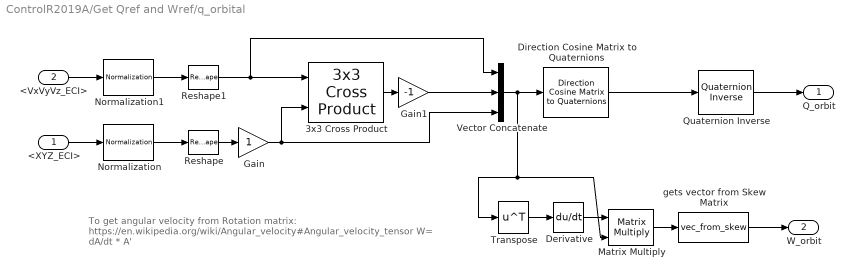
== system ControlR2019A/Get Qref and Wref/q_orbital ==
  note: To get angular velocity from Rotation matrix:
      | https://en.wikipedia.org/wiki/Angular_velocity#Angular_velocity_tensor
      | W= dA/dt * A'
  <XYZ_ECI> : Inport
  <VxVyVz_ECI> : Inport  Port=2
  3x3 Cross Product : sharedutil/3x3 Cross Product  aMode=aMode
      settings: SourceProductBaseCode=AE,PW,MT,UV,VE,VP
  Derivative : Derivative
  Direction Cosine Matrix to Quaternions : sharedtransform/Direction Cosine Matrix  to Quaternions  aMode=0  action=None  tolerance=eps(2)
      settings: SourceProductBaseCode=AE,PW,MT,UV,VE,VP
  Gain : Gain
  Gain1 : Gain  Gain=-1
  Matrix Multiply : Product  Multiplication=Matrix(*)
  Normalization : dspmathops/Normalization  NormType=2-norm  Bias=1e-10  NormOver=Each column  Dimension=1  roundingMode=Floor  overflowMode=off  accumDataTypeStr=Inherit: Same as product output  accumLastDataTypeStr=Inherit: Same as product output  outputDataTypeStr=Inherit: Same as product output  outputMin=[]  outputMax=[]  outputLastDataTypeStr=Inherit: Same as product output
  Normalization1 : dspmathops/Normalization  NormType=2-norm  Bias=1e-10  NormOver=Each column  Dimension=1  roundingMode=Floor  overflowMode=off  accumDataTypeStr=Inherit: Same as product output  accumLastDataTypeStr=Inherit: Same as product output  outputDataTypeStr=Inherit: Same as product output  outputMin=[]  outputMax=[]  outputLastDataTypeStr=Inherit: Same as product output
  Quaternion Inverse : aerolibutil/Quaternion Inverse
  Reshape : Reshape  OutputDimensionality=Column vector (2-D)
  Reshape1 : Reshape  OutputDimensionality=Column vector (2-D)
  Transpose : Math  Operator=transpose  SaturateOnIntegerOverflow=on
  Vector Concatenate : Concatenate  NumInputs=3  Mode=Multidimensional array  ConcatenateDimension=2
  gets vector from Skew Matrix : MATLABFcn  MATLABFcn=vec_from_skew
  Q_orbit : Outport  VectorParamsAs1DForOutWhenUnconnected=off
  W_orbit : Outport  Port=2
  wires:
  Normalization/1 -> Reshape/1
  Normalization1/1 -> Reshape1/1
  <VxVyVz_ECI>/1 -> Normalization1/1
  Reshape1/1 -> 3x3 Cross Product/1, Vector Concatenate/1
  <XYZ_ECI>/1 -> Normalization/1
  Reshape/1 -> Gain/1
  Gain/1 -> 3x3 Cross Product/2, Vector Concatenate/3
  Direction Cosine Matrix to Quaternions/1 -> Quaternion Inverse/1
  3x3 Cross Product/1 -> Gain1/1
  Gain1/1 -> Vector Concatenate/2
  Quaternion Inverse/1 -> Q_orbit/1
  Vector Concatenate/1 -> Transpose/1, Matrix Multiply/2, Direction Cosine Matrix to Quaternions/1
  Derivative/1 -> Matrix Multiply/1
  gets vector from Skew Matrix/1 -> W_orbit/1
  Matrix Multiply/1 -> gets vector from Skew Matrix/1
  Transpose/1 -> Derivative/1

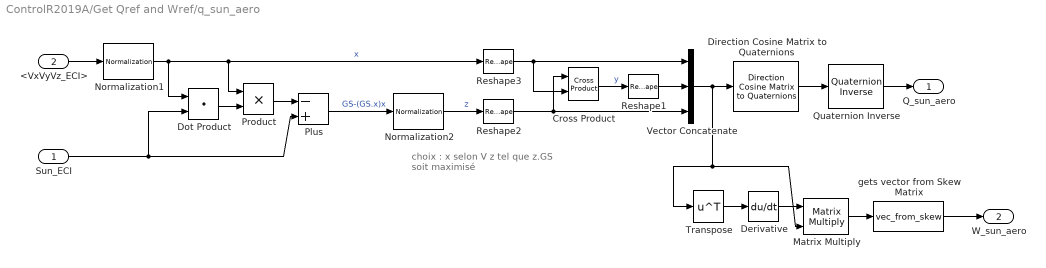
== system ControlR2019A/Get Qref and Wref/q_sun_aero ==
  note: choix :
      | x selon V
      | z tel que z.GS soit maximisé
  Sun_ECI : Inport
  <VxVyVz_ECI> : Inport  Port=2
  Cross Product : vrlib/Utilities/Cross Product
  Derivative : Derivative
  Direction Cosine Matrix to Quaternions : sharedtransform/Direction Cosine Matrix  to Quaternions  aMode=0  action=None  tolerance=eps(2)
      settings: SourceProductBaseCode=AE,PW,MT,UV,VE,VP
  Dot Product : DotProduct  InputSameDT=on  OutDataTypeStr=Inherit: Inherit via internal rule
  Matrix Multiply : Product  Multiplication=Matrix(*)
  Normalization1 : dspmathops/Normalization  NormType=2-norm  Bias=1e-10  NormOver=Each column  Dimension=1  roundingMode=Floor  overflowMode=off  accumDataTypeStr=Inherit: Same as product output  accumLastDataTypeStr=Inherit: Same as product output  outputDataTypeStr=Inherit: Same as product output  outputMin=[]  outputMax=[]  outputLastDataTypeStr=Inherit: Same as product output
  Normalization2 : dspmathops/Normalization  NormType=2-norm  Bias=1e-10  NormOver=Each column  Dimension=1  roundingMode=Floor  overflowMode=off  accumDataTypeStr=Inherit: Same as product output  accumLastDataTypeStr=Inherit: Same as product output  outputDataTypeStr=Inherit: Same as product output  outputMin=[]  outputMax=[]  outputLastDataTypeStr=Inherit: Same as product output
  Plus : Sum  Inputs=-+
  Product : Product
  Quaternion Inverse : aerolibutil/Quaternion Inverse
  Reshape1 : Reshape  OutputDimensionality=Column vector (2-D)
  Reshape2 : Reshape  OutputDimensionality=Column vector (2-D)
  Reshape3 : Reshape  OutputDimensionality=Column vector (2-D)
  Transpose : Math  Operator=transpose  SaturateOnIntegerOverflow=on
  Vector Concatenate : Concatenate  NumInputs=3  Mode=Multidimensional array  ConcatenateDimension=2
  gets vector from Skew Matrix : MATLABFcn  MATLABFcn=vec_from_skew
  Q_sun_aero : Outport  VectorParamsAs1DForOutWhenUnconnected=off
  W_sun_aero : Outport  Port=2
  wires:
  Quaternion Inverse/1 -> Q_sun_aero/1
  Reshape2/1 -> Cross Product/1, Vector Concatenate/3
  Reshape3/1 -> Vector Concatenate/1, Cross Product/2
  Product/1 -> Plus/1
  Dot Product/1 -> Product/2
  Cross Product/1 -> Reshape1/1  "y"
  Normalization2/1 -> Reshape2/1  "z"
  Plus/1 -> Normalization2/1  "GS-(GS.x)x"
  Sun_ECI/1 -> Dot Product/2, Plus/2
  Direction Cosine Matrix to Quaternions/1 -> Quaternion Inverse/1
  Normalization1/1 -> Dot Product/1, Product/1, Reshape3/1  "x"
  <VxVyVz_ECI>/1 -> Normalization1/1
  Reshape1/1 -> Vector Concatenate/2
  Matrix Multiply/1 -> gets vector from Skew Matrix/1
  Derivative/1 -> Matrix Multiply/1
  Transpose/1 -> Derivative/1
  Vector Concatenate/1 -> Transpose/1, Matrix Multiply/2, Direction Cosine Matrix to Quaternions/1
  gets vector from Skew Matrix/1 -> W_sun_aero/1

== system ControlR2019A/IGRF Computation block/Obtain B_ECI ==
  In1 : Inport
  Dipole Subsystem : Subsystem  TreatAsAtomicUnit=on
  IGRF Subsystem : Subsystem  TreatAsAtomicUnit=on
  If : If
  Merge : Merge
  Use_IGRF : Constant  Value=Use_IGRF
  Out1 : Outport  VectorParamsAs1DForOutWhenUnconnected=off
  wires:
  If/1 -> IGRF Subsystem/Action
  In1/1 -> Dipole Subsystem/1(In1), IGRF Subsystem/1(In1)
  IGRF Subsystem/1(Out1) -> Merge/1
  Use_IGRF/1 -> If/1
  Merge/1 -> Out1/1
  Dipole Subsystem/1("B_ECI ") -> Merge/2
  If/2 -> Dipole Subsystem/Action

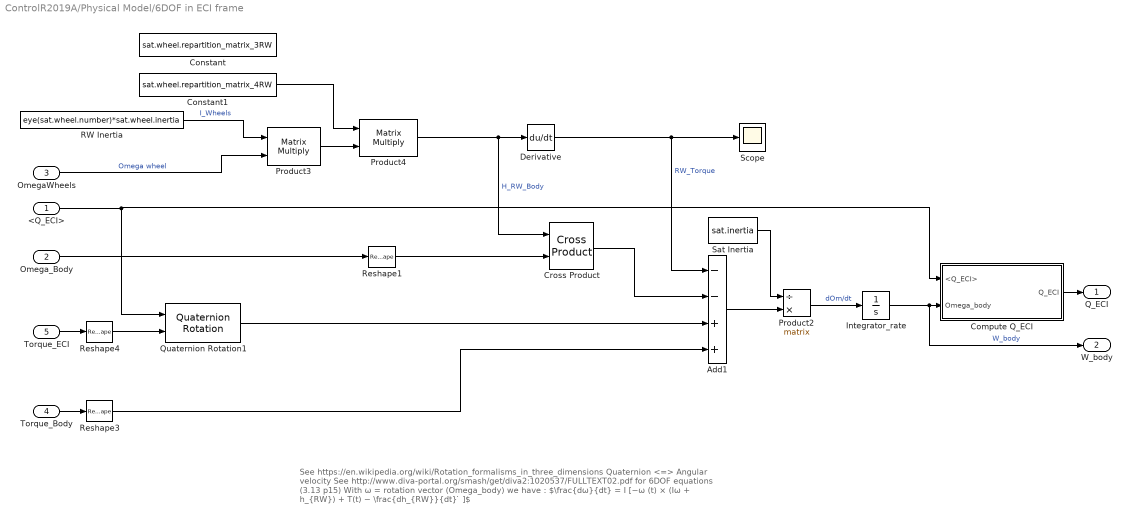
== system ControlR2019A/Physical Model/6DOF in ECI frame ==
  note: See https://en.wikipedia.org/wiki/Rotation_formalisms_in_three_dimensions Quaternion <=> Angular velocity
      |
      | See http://www.diva-portal.org/smash/get/diva2:1020537/FULLTEXT02.pdf for 6DOF equations (3.13 p15)
      |
      | With ω = rotation vector (Omega_body) we have :
      |
      | $\frac{dω}{dt} = I [−ω (t) × (Iω + h_{RW}) + T(t) − \frac{dh_{RW}}{dt} ̇ ]$
  <Q_ECI> : Inport
  "Omega_Body " : Inport  Port=2
  OmegaWheels : Inport  Port=3
  Torque_Body : Inport  Port=4
  Torque_ECI : Inport  Port=5  PortDimensions=3
  Add1 : Sum  Inputs=--++
  Compute Q_ECI : Subsystem
  Constant : Constant  Value=sat.wheel.repartition_matrix_3RW
  Constant1 : Constant  Value=sat.wheel.repartition_matrix_4RW
  Cross Product : vrlib/Utilities/Cross Product
  Derivative : Derivative
  Integrator_rate : Integrator
  Product2 : Product  Inputs=/*  Multiplication=Matrix(*)
  Product3 : Product  Multiplication=Matrix(*)
  Product4 : Product  Multiplication=Matrix(*)
  Quaternion Rotation1 : aerolibutil/Quaternion Rotation
  RW Inertia : Constant  Value=eye(sat.wheel.number)*sat.wheel.inertia
  Reshape1 : Reshape  OutputDimensionality=Column vector (2-D)
  Reshape3 : Reshape  OutputDimensionality=Column vector (2-D)
  Reshape4 : Reshape  OutputDimensionality=Column vector (2-D)
  Sat Inertia : Constant  Value=sat.inertia
  Scope : Scope
  Q_ECI : Outport  VectorParamsAs1DForOutWhenUnconnected=off
  W_body : Outport  Port=2  VectorParamsAs1DForOutWhenUnconnected=off
  wires:
  Product2/1 -> Integrator_rate/1  "dOm/dt"
  Product3/1 -> Product4/2
  Sat Inertia/1 -> Product2/1
  Add1/1 -> Product2/2
  Cross Product/1 -> Add1/2
  "Omega_Body "/1 -> Reshape1/1
  Integrator_rate/1 -> W_body/1, Compute Q_ECI/2(Omega_body)  "W_body"
  RW Inertia/1 -> Product3/1  "I_Wheels"
  Torque_Body/1 -> Reshape3/1
  Derivative/1 -> Scope/1, Add1/1  "RW_Torque"
  OmegaWheels/1 -> Product3/2  "Omega wheel"
  Compute Q_ECI/1(Q_ECI) -> Q_ECI/1
  Torque_ECI/1 -> Reshape4/1
  <Q_ECI>/1 -> Quaternion Rotation1/1, Compute Q_ECI/1(<Q_ECI>)
  Quaternion Rotation1/1 -> Add1/3
  Constant1/1 -> Product4/1
  Reshape3/1 -> Add1/4
  Reshape4/1 -> Quaternion Rotation1/2
  Product4/1 -> Cross Product/1, Derivative/1  "H_RW_Body"
  Reshape1/1 -> Cross Product/2

== system ControlR2019A/Physical Model/Magnetorquer physics ==
  note: On pourrait aussi changer les blocs
      | magnétocoupleurs pour sortir les intensités
  Mag vector command : Inport
  B_IGRF_body (vecteur) : Inport  Port=2
  Add1 : Sum  Inputs=+++
  Cross Product : vrlib/Utilities/Cross Product
  Demux : Demux  Outputs=3
  Magnétocoupleur 1 : Subsystem
  Magnétocoupleur 2 : Subsystem
  Magnétocoupleur 3 : Subsystem
  Couple (vect) : Outport  PortDimensions=3  VectorParamsAs1DForOutWhenUnconnected=off
  Real mag moments vector : Outport  Port=2  VectorParamsAs1DForOutWhenUnconnected=off
  wires:
  Add1/1 -> Real mag moments vector/1, Cross Product/1  "M_real"
  Demux/1 -> Magnétocoupleur 1/1(m_in (scalar))
  Demux/2 -> Magnétocoupleur 2/1(m_in (scalar))
  Demux/3 -> Magnétocoupleur 3/1(m_in (scalar))
  Mag vector command/1 -> Demux/1
  Magnétocoupleur 2/1(m_out (vect)) -> Add1/2
  Magnétocoupleur 1/1(m_out (vect)) -> Add1/1
  Magnétocoupleur 3/1(m_out (vect)) -> Add1/3
  Cross Product/1 -> Couple (vect)/1  "T_body"
  B_IGRF_body (vecteur)/1 -> Cross Product/2

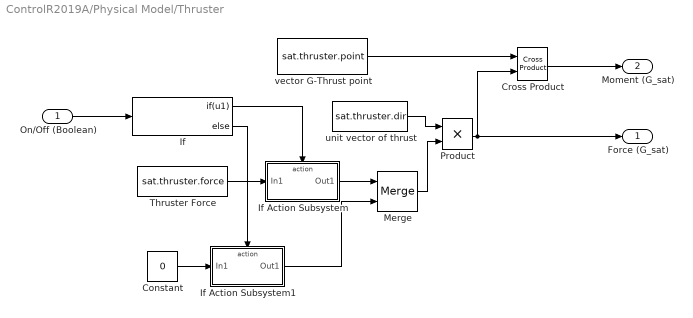
== system ControlR2019A/Physical Model/Thruster ==
  On/Off (Boolean) : Inport  OutDataTypeStr=boolean
  Constant : Constant  Value=0
  Cross Product : vrlib/Utilities/Cross Product
  If : If  IfExpression=u1
  If Action Subsystem : Subsystem  TreatAsAtomicUnit=on
  If Action Subsystem1 : Subsystem  TreatAsAtomicUnit=on
  Merge : Merge
  Product : Product
  Thruster Force : Constant  Value=sat.thruster.force
  unit vector of thrust : Constant  Value=sat.thruster.dir
  vector G-Thrust point : Constant  Value=sat.thruster.point
  Force (G_sat) : Outport  VectorParamsAs1DForOutWhenUnconnected=off
  Moment (G_sat) : Outport  Port=2  VectorParamsAs1DForOutWhenUnconnected=off
  wires:
  Product/1 -> Force (G_sat)/1, Cross Product/2
  vector G-Thrust point/1 -> Cross Product/1
  unit vector of thrust/1 -> Product/1
  Cross Product/1 -> Moment (G_sat)/1
  Thruster Force/1 -> If Action Subsystem/1(In1)
  On/Off (Boolean)/1 -> If/1
  If/1 -> If Action Subsystem/Action
  If/2 -> If Action Subsystem1/Action
  If Action Subsystem1/1(Out1) -> Merge/2
  If Action Subsystem/1(Out1) -> Merge/1
  Merge/1 -> Product/2
  Constant/1 -> If Action Subsystem1/1(In1)

== system ControlR2019A/Attitude Controller/Magnetorquer Magnetic Momend Command/Switch Case Action Subsystem3 ==
  In1 : Inport
  Action Port : ActionPort
  Out1 : Outport  VectorParamsAs1DForOutWhenUnconnected=off
  wires:
  In1/1 -> Out1/1

== system ControlR2019A/Attitude Controller/Magnetorquer Magnetic Momend Command/Switch Case Action Subsystem4 ==
  In1 : Inport
  Action Port : ActionPort
  Out1 : Outport  VectorParamsAs1DForOutWhenUnconnected=off
  wires:
  In1/1 -> Out1/1

== system ControlR2019A/Attitude Controller/PID (nominal command)/Command Magnetic moments computation ==
  note: Moment magnétique de commande M :
      |
      | $M_c = \frac{1}{B²}\vec{B} \wedge\vec{T_P}$
      |
      | Avec Tp couple projeté dans le plan orthogonal à B
      | $T_P=\vec{T}-\frac{1}{B²}(\vec{T}\cdot\vec{B})\vec{B}$
  Command (vect) : Inport  OutDataTypeStr=double
  B_IGRF_body (vect) : Inport  Port=2  OutDataTypeStr=double
  h1 (vect) : Inport  Port=3
  h2 (vect) : Inport  Port=4
  h3 (vect) : Inport  Port=5
  Cross Product : vrlib/Utilities/Cross Product
  Dot Product : DotProduct  InputSameDT=on  OutDataTypeStr=Inherit: Inherit via internal rule
  Global magnetic moment computation : Subsystem
  Mux : Mux  Inputs=3
  Product1 : Product  Inputs=*/
  Reshape : Reshape  OutputDimensionality=Column vector (2-D)
  Reshape1 : Reshape  OutputDimensionality=Column vector (2-D)
  Mag vector command : Outport  VectorParamsAs1DForOutWhenUnconnected=off
  wires:
  B_IGRF_body (vect)/1 -> Reshape1/1  "B_Body"
  Command (vect)/1 -> Reshape/1  "T_Body"
  h1 (vect)/1 -> Global magnetic moment computation/2(In2)
  h2 (vect)/1 -> Global magnetic moment computation/3(In3)
  h3 (vect)/1 -> Global magnetic moment computation/4(In4)
  Global magnetic moment computation/2(magnetic moment 2 (scalar)) -> Mux/2  "magnetic moment 2"
  Global magnetic moment computation/3(magnetic moment 3 (scalar)) -> Mux/3  "magnetic moment 3"
  Global magnetic moment computation/1(magnetic moment 1 (scalar)) -> Mux/1  "magnetic moment 1"
  Mux/1 -> Mag vector command/1
  Reshape1/1 -> Cross Product/2, Dot Product/2, Dot Product/1
  Cross Product/1 -> Product1/1
  Product1/1 -> Global magnetic moment computation/1(In1)  "Mc"
  Dot Product/1 -> Product1/2  "B^2"
  Reshape/1 -> Cross Product/1  "Tp"

== system ControlR2019A/Attitude Controller/PID (nominal command)/Extract Vect ==
  Qr : Inport
  Demux : Demux
  Mux1 : Mux  Inputs=3
  Product : Product
  Reshape : Reshape  OutputDimensionality=Column vector (2-D)
  Sign : Signum
  Qvect : Outport  VectorParamsAs1DForOutWhenUnconnected=off
  wires:
  Demux/2 -> Mux1/1
  Demux/4 -> Mux1/3
  Demux/3 -> Mux1/2
  Demux/1 -> Sign/1
  Qr/1 -> Demux/1
  Mux1/1 -> Product/2
  Product/1 -> Reshape/1
  Sign/1 -> Product/1
  Reshape/1 -> Qvect/1

== system ControlR2019A/Attitude Controller/PID (nominal command)/If Action Subsystem ==
  In1 : Inport
  Action Port : ActionPort
  Out1 : Outport  VectorParamsAs1DForOutWhenUnconnected=off
  wires:
  In1/1 -> Out1/1

== system ControlR2019A/Attitude Controller/PID (nominal command)/If Action Subsystem1 ==
  In1 : Inport
  Action Port : ActionPort
  Out1 : Outport  VectorParamsAs1DForOutWhenUnconnected=off
  wires:
  In1/1 -> Out1/1

== system ControlR2019A/Attitude Controller/PID (nominal command)/If Action Subsystem2 ==
  In1 : Inport
  Action Port : ActionPort
  Out1 : Outport  VectorParamsAs1DForOutWhenUnconnected=off
  wires:
  In1/1 -> Out1/1

== system ControlR2019A/Attitude Controller/PID (nominal command)/If Action Subsystem3 ==
  In1 : Inport
  Action Port : ActionPort
  Out1 : Outport  VectorParamsAs1DForOutWhenUnconnected=off
  wires:
  In1/1 -> Out1/1

== system ControlR2019A/Attitude Controller/PID (nominal command)/RW1 ==
  note: Entrées:
      | - Moment de commande (déjà projeté sur l'axe de la roue...)
      | Sorties:
      | - Omega de commande à appliquer
  Mc (scalar) : Inport
  Discrete-Time Integrator : DiscreteIntegrator  IntegratorMethod=Integration: Trapezoidal  SampleTime=-1  ICPrevOutput=DiscIntNeverNeededParam  ICPrevScaledInput=DiscIntNeverNeededParam
  Divide : Product  Inputs=*/
  Saturation_speed : Saturate  UpperLimit=sat.wheel.max_speed  LowerLimit=- sat.wheel.max_speed
  Torque_sat : Saturate  UpperLimit=sat.wheel.max_torque  LowerLimit=- sat.wheel.max_torque
  Wheel Inertia : Constant  Value=sat.wheel.max_sigma/sat.wheel.max_speed
  Omega_C (scalar) : Outport
  wires:
  Wheel Inertia/1 -> Divide/2
  Divide/1 -> Discrete-Time Integrator/1  "dw/dt"
  Discrete-Time Integrator/1 -> Saturation_speed/1
  Torque_sat/1 -> Divide/1  "Torque (scal)"
  Saturation_speed/1 -> Omega_C (scalar)/1
  Mc (scalar)/1 -> Torque_sat/1

== system ControlR2019A/Attitude Controller/PID (nominal command)/RW2 ==
  note: Entrées:
      | - Moment de commande (déjà projeté sur l'axe de la roue...)
      | Sorties:
      | - Omega de commande à appliquer
  Mc (scalar) : Inport
  Discrete-Time Integrator : DiscreteIntegrator  IntegratorMethod=Integration: Trapezoidal  SampleTime=-1  ICPrevOutput=DiscIntNeverNeededParam  ICPrevScaledInput=DiscIntNeverNeededParam
  Divide : Product  Inputs=*/
  Saturation_speed : Saturate  UpperLimit=sat.wheel.max_speed  LowerLimit=- sat.wheel.max_speed
  Torque_sat : Saturate  UpperLimit=sat.wheel.max_torque  LowerLimit=- sat.wheel.max_torque
  Wheel Inertia : Constant  Value=sat.wheel.max_sigma/sat.wheel.max_speed
  Omega_C (scalar) : Outport
  wires:
  Wheel Inertia/1 -> Divide/2
  Divide/1 -> Discrete-Time Integrator/1  "dw/dt"
  Discrete-Time Integrator/1 -> Saturation_speed/1
  Torque_sat/1 -> Divide/1  "Torque (scal)"
  Saturation_speed/1 -> Omega_C (scalar)/1
  Mc (scalar)/1 -> Torque_sat/1

== system ControlR2019A/Attitude Controller/PID (nominal command)/RW3 ==
  note: Entrées:
      | - Moment de commande (déjà projeté sur l'axe de la roue...)
      | Sorties:
      | - Omega de commande à appliquer
  Mc (scalar) : Inport
  Discrete-Time Integrator : DiscreteIntegrator  IntegratorMethod=Integration: Trapezoidal  SampleTime=-1  ICPrevOutput=DiscIntNeverNeededParam  ICPrevScaledInput=DiscIntNeverNeededParam
  Divide : Product  Inputs=*/
  Saturation_speed : Saturate  UpperLimit=sat.wheel.max_speed  LowerLimit=- sat.wheel.max_speed
  Torque_sat : Saturate  UpperLimit=sat.wheel.max_torque  LowerLimit=- sat.wheel.max_torque
  Wheel Inertia : Constant  Value=sat.wheel.max_sigma/sat.wheel.max_speed
  Omega_C (scalar) : Outport
  wires:
  Wheel Inertia/1 -> Divide/2
  Divide/1 -> Discrete-Time Integrator/1  "dw/dt"
  Discrete-Time Integrator/1 -> Saturation_speed/1
  Torque_sat/1 -> Divide/1  "Torque (scal)"
  Saturation_speed/1 -> Omega_C (scalar)/1
  Mc (scalar)/1 -> Torque_sat/1

== system ControlR2019A/Attitude Controller/PID (nominal command)/RW4  ==
  note: Entrées:
      | - Moment de commande (déjà projeté sur l'axe de la roue...)
      | Sorties:
      | - Omega de commande à appliquer
  Mc (scalar) : Inport
  Discrete-Time Integrator : DiscreteIntegrator  IntegratorMethod=Integration: Trapezoidal  SampleTime=-1  ICPrevOutput=DiscIntNeverNeededParam  ICPrevScaledInput=DiscIntNeverNeededParam
  Divide : Product  Inputs=*/
  Saturation_speed : Saturate  UpperLimit=sat.wheel.max_speed  LowerLimit=- sat.wheel.max_speed
  Torque_sat : Saturate  UpperLimit=sat.wheel.max_torque  LowerLimit=- sat.wheel.max_torque
  Wheel Inertia : Constant  Value=sat.wheel.max_sigma/sat.wheel.max_speed
  Omega_C (scalar) : Outport
  wires:
  Wheel Inertia/1 -> Divide/2
  Divide/1 -> Discrete-Time Integrator/1  "dw/dt"
  Discrete-Time Integrator/1 -> Saturation_speed/1
  Torque_sat/1 -> Divide/1  "Torque (scal)"
  Saturation_speed/1 -> Omega_C (scalar)/1
  Mc (scalar)/1 -> Torque_sat/1

== system ControlR2019A/Attitude Controller/Reaction Wheels Speed Command/Switch Case Action Subsystem3 ==
  In1 : Inport
  Action Port : ActionPort
  Out1 : Outport  VectorParamsAs1DForOutWhenUnconnected=off
  wires:
  In1/1 -> Out1/1

== system ControlR2019A/Attitude Controller/Reaction Wheels Speed Command/Switch Case Action Subsystem4 ==
  In1 : Inport
  Action Port : ActionPort
  Out1 : Outport  VectorParamsAs1DForOutWhenUnconnected=off
  wires:
  In1/1 -> Out1/1

== system ControlR2019A/IGRF Computation block/Obtain B_ECI/Dipole Subsystem ==
  In1 : Inport
  Action Port : ActionPort
  Bus Selector1 : BusSelector  OutputSignals=h,lat,long,DCM_i2e
  Dipole Model : Subsystem  AncestorBlock=DipoleModel/Dipole Model
  "B_ECI " : Outport  VectorParamsAs1DForOutWhenUnconnected=off
  wires:
  In1/1 -> Bus Selector1/1
  Bus Selector1/1 -> Dipole Model/1(h)  "<h>"
  Bus Selector1/2 -> Dipole Model/2("lat ")  "<lat>"
  Bus Selector1/3 -> Dipole Model/3(long)  "<long>"
  Bus Selector1/4 -> Dipole Model/4(ECI2ECEF_DCM)  "<DCM_i2e>"
  Dipole Model/1("B_ECI ") -> "B_ECI "/1
